simulink model "FIRCoeffCalc"  (R2019a)
settings: Solver=VariableStepAuto  StartTime=0.0  StopTime=(nSamp - 1)*Ts  RelTol=1e-3
InitFcn:
  | block_verScript;
values from neighbouring files (symbols this model uses):
  Ts = 1/Fs    (= 2.08333333333e-05)    [FIR_filterTestm.m]    (also in JMAP_INIT.m; blockVerification.m; block_verScript.m; ksi_verScript.m)
undefined symbols (not defined in the file or in its folder): magnitude
libraries: simulink x1
settings Model: Creator=Showi  LastModifiedBy=Showi

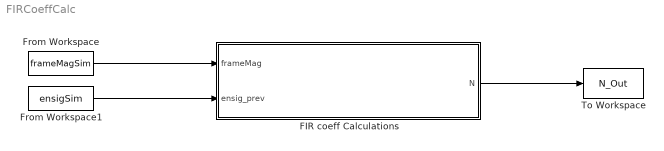
== system FIRCoeffCalc ==
  FIR coeff Calculations : Subsystem
  From Workspace : FromWorkspace  VariableName=frameMagSim  SampleTime=Ts
  From Workspace1 : FromWorkspace  VariableName=ensigSim  SampleTime=Ts
  To Workspace : ToWorkspace  VariableName=N_Out  SaveFormat=Timeseries  SampleTime=-1
  wires:
  From Workspace/1 -> FIR coeff Calculations/1(frameMag)
  From Workspace1/1 -> FIR coeff Calculations/2(ensig_prev)
  FIR coeff Calculations/1(N) -> To Workspace/1

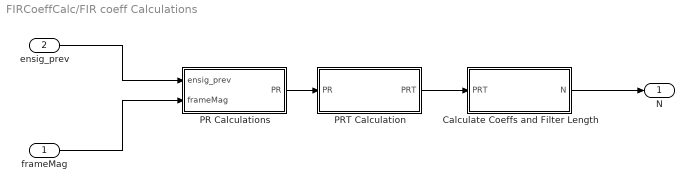
== system FIRCoeffCalc/FIR coeff Calculations ==
  frameMag : Inport
  ensig_prev : Inport  Port=2
  Calculate Coeffs and Filter Length : Subsystem
  PR Calculations : Subsystem
  PRT Calculation : Subsystem
  N : Outport
  wires:
  ensig_prev/1 -> PR Calculations/1(ensig_prev)
  PR Calculations/1(PR) -> PRT Calculation/1(PR)
  Calculate Coeffs and Filter Length/1(N) -> N/1
  PRT Calculation/1(PRT) -> Calculate Coeffs and Filter Length/1(PRT)
  frameMag/1 -> PR Calculations/2(frameMag)

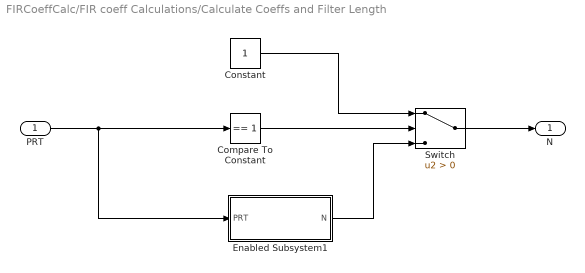
== system FIRCoeffCalc/FIR coeff Calculations/Calculate Coeffs and Filter Length ==
  PRT : Inport
  Compare To Constant : simulink/Logic and Bit Operations/Compare To Constant  relop===  const=1  OutDataTypeStr=boolean
  Constant : Constant  SampleTime=-1
  Enabled Subsystem1 : Subsystem  TreatAsAtomicUnit=on
  Switch : Switch  Criteria=u2 > Threshold
  N : Outport
  wires:
  PRT/1 -> Compare To Constant/1, Enabled Subsystem1/1(PRT)
  Compare To Constant/1 -> Switch/2
  Constant/1 -> Switch/1
  Enabled Subsystem1/1(N) -> Switch/3
  Switch/1 -> N/1

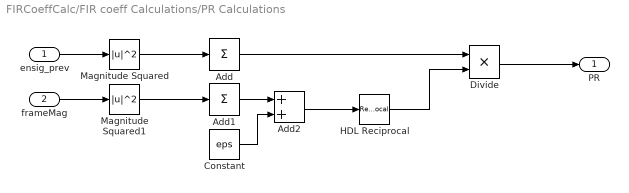
== system FIRCoeffCalc/FIR coeff Calculations/PR Calculations ==
  ensig_prev : Inport
  frameMag : Inport  Port=2
  Add : Sum  Inputs=+
  Add1 : Sum  Inputs=+
  Add2 : Sum
  Constant : Constant  Value=eps  SampleTime=-1
  Divide : Product  Inputs=**  SaturateOnIntegerOverflow=on  RndMeth=Zero
  HDL Reciprocal : Reciprocal
  Magnitude Squared : Math  Operator=magnitude^2  SaturateOnIntegerOverflow=on
  Magnitude Squared1 : Math  Operator=magnitude^2  SaturateOnIntegerOverflow=on
  PR : Outport
  wires:
  Magnitude Squared/1 -> Add/1
  ensig_prev/1 -> Magnitude Squared/1
  Add/1 -> Divide/1
  Magnitude Squared1/1 -> Add1/1
  frameMag/1 -> Magnitude Squared1/1
  Add1/1 -> Add2/1
  Constant/1 -> Add2/2
  Add2/1 -> HDL Reciprocal/1
  Divide/1 -> PR/1
  HDL Reciprocal/1 -> Divide/2

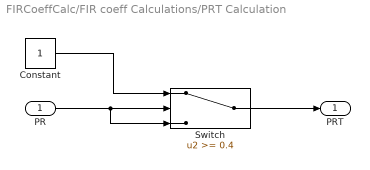
== system FIRCoeffCalc/FIR coeff Calculations/PRT Calculation ==
  PR : Inport
  Constant : Constant  SampleTime=-1
  Switch : Switch  Threshold=0.4
  PRT : Outport
  wires:
  PR/1 -> Switch/3, Switch/2
  Constant/1 -> Switch/1
  Switch/1 -> PRT/1

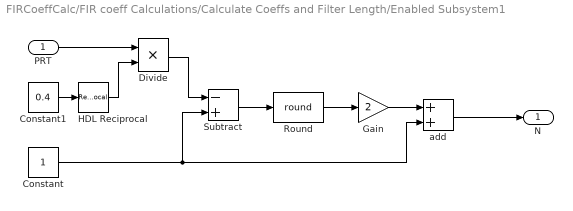
== system FIRCoeffCalc/FIR coeff Calculations/Calculate Coeffs and Filter Length/Enabled Subsystem1 ==
  PRT : Inport
  Constant : Constant  SampleTime=-1
  Constant1 : Constant  Value=0.4  SampleTime=-1
  Divide : Product  Inputs=**  SaturateOnIntegerOverflow=on  RndMeth=Zero
  Gain : Gain  Gain=2
  HDL Reciprocal : Reciprocal
  Round : Rounding  Operator=round
  Subtract : Sum  Inputs=-+
  add : Sum
  N : Outport  InitialOutput=0
  wires:
  Gain/1 -> add/1
  PRT/1 -> Divide/1
  Constant/1 -> add/2, Subtract/2
  Subtract/1 -> Round/1
  Constant1/1 -> HDL Reciprocal/1
  Divide/1 -> Subtract/1
  Round/1 -> Gain/1
  add/1 -> N/1
  HDL Reciprocal/1 -> Divide/2
